simulink model "modellqrN1"  (R2023b)
settings: Solver=VariableStepAuto  StartTime=0.0  StopTime=1000  FixedStep=0.0001  MaxStep=1  MinStep=0.1  RelTol=1e-3
values from neighbouring files (symbols this model uses):
  g_ = 9.81    [main.m]
  h1_ = 0.15    [main.m]
  h2_ = (a^2*h1_)/(b^2)    [main.m]
  K = lqr(A,B,Q,R)    [main.m]
  N = 1/([0 1] *(-inv(A-B.*K'))* B)    [main.m]
  p1_ = 0.85    [main.m]
  p2_ = 0.95    [main.m]
  q0_ = a*sqrt(h1_)    [main.m]
  s1_ = 0.083    [main.m]
  S1_ = 2*pi*R1_*h1_ + 2*pi*R1_^2    (= 27.0176968209)    [main.m]
  s2_ = 0.083    [main.m]
  S2_ = 2*pi*R2_*h2_ + 2*pi*R2_^2    [main.m]
settings Model: Creator=ralex  LastModifiedBy=ralex

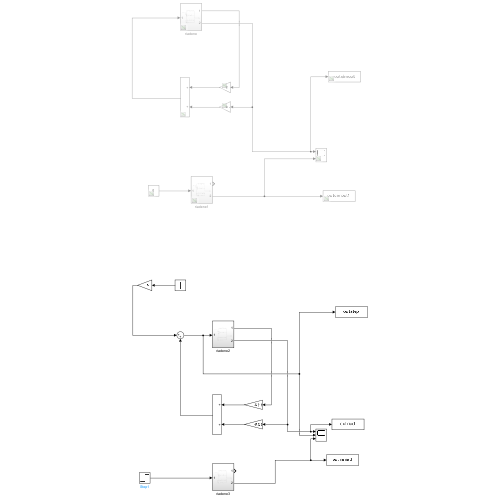
[thumbnail: Simulink's stored preview of the top-level diagram]
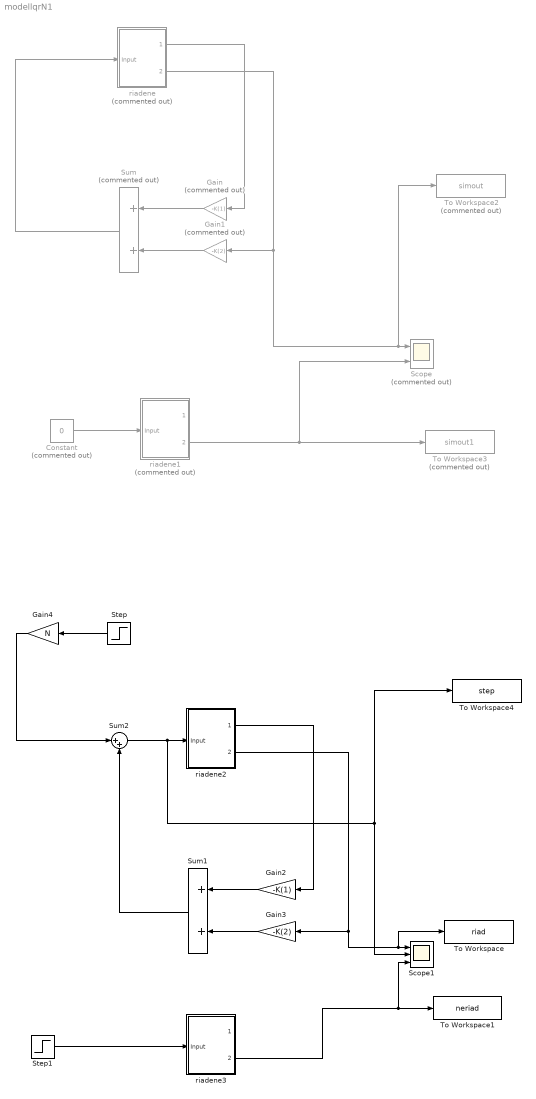
== system modellqrN1 ==
  Constant : Constant  Commented=on  Value=0
  Gain : Gain  Commented=on  Gain=-K(1)
  Gain1 : Gain  Commented=on  Gain=-K(2)
  Gain2 : Gain  Gain=-K(1)
  Gain3 : Gain  Gain=-K(2)
  Gain4 : Gain  Gain=N
  Scope : Scope  Commented=on  NumInputPorts=2
  Scope1 : Scope  NumInputPorts=3
  Step : Step  Time=100  After=h2_  SampleTime=0
  Step1 : Step  Time=100  After=q0_  SampleTime=0
  Sum : Sum  Commented=on
  Sum1 : Sum
  Sum2 : Sum  Inputs=|++
  To Workspace : ToWorkspace  VariableName=riad  SaveFormat=Timeseries  SampleTime=-1
  To Workspace1 : ToWorkspace  VariableName=neriad  SaveFormat=Timeseries  SampleTime=-1
  To Workspace2 : ToWorkspace  Commented=on  VariableName=simout  SaveFormat=Timeseries  SampleTime=-1
  To Workspace3 : ToWorkspace  Commented=on  VariableName=simout1  SaveFormat=Timeseries  SampleTime=-1
  To Workspace4 : ToWorkspace  VariableName=step  SaveFormat=Timeseries  SampleTime=-1
  riadene : Subsystem  Commented=on
  riadene1 : Subsystem  Commented=on
  riadene2 : Subsystem
  riadene3 : Subsystem
  wires:
  riadene/2(Output) -> To Workspace2/1, Scope/1, Gain1/1
  riadene/1(Output1) -> Gain/1
  Gain1/1 -> Sum/2
  Gain/1 -> Sum/1
  Sum/1 -> riadene/1(Input)
  Constant/1 -> riadene1/1(Input)
  riadene1/2(Output) -> To Workspace3/1, Scope/2
  Gain2/1 -> Sum1/1
  Gain3/1 -> Sum1/2
  Step/1 -> Gain4/1
  Sum2/1 -> To Workspace4/1, Scope1/2, riadene2/1(Input)
  Sum1/1 -> Sum2/2
  Gain4/1 -> Sum2/1
  riadene2/2(Output) -> To Workspace/1, Scope1/1, Gain3/1
  riadene2/1(Output1) -> Gain2/1
  riadene3/2(Output) -> Scope1/3, To Workspace1/1
  Step1/1 -> riadene3/1(Input)

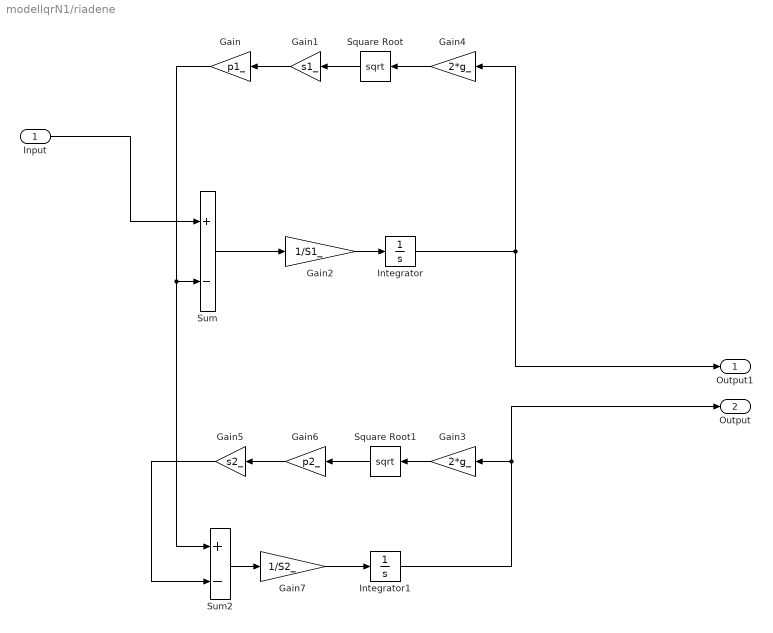
== system modellqrN1/riadene ==
  Input : Inport
  Gain : Gain  Gain=p1_
  Gain1 : Gain  Gain=s1_
  Gain2 : Gain  Gain=1/S1_
  Gain3 : Gain  Gain=2*g_
  Gain4 : Gain  Gain=2*g_
  Gain5 : Gain  Gain=s2_
  Gain6 : Gain  Gain=p2_
  Gain7 : Gain  Gain=1/S2_
  Integrator : Integrator  InitialCondition=h1_
  Integrator1 : Integrator  InitialCondition=h2_
  Square Root : Sqrt
  Square Root1 : Sqrt
  Sum : Sum  Inputs=+-
  Sum2 : Sum  Inputs=+-
  Output1 : Outport
  Output : Outport  Port=2
  wires:
  Gain/1 -> Sum/2, Sum2/1
  Gain1/1 -> Gain/1
  Input/1 -> Sum/1
  Integrator/1 -> Output1/1, Gain4/1
  Square Root/1 -> Gain1/1
  Gain4/1 -> Square Root/1
  Gain5/1 -> Sum2/2
  Sum/1 -> Gain2/1
  Integrator1/1 -> Output/1, Gain3/1
  Gain6/1 -> Gain5/1
  Square Root1/1 -> Gain6/1
  Gain3/1 -> Square Root1/1
  Sum2/1 -> Gain7/1
  Gain2/1 -> Integrator/1
  Gain7/1 -> Integrator1/1

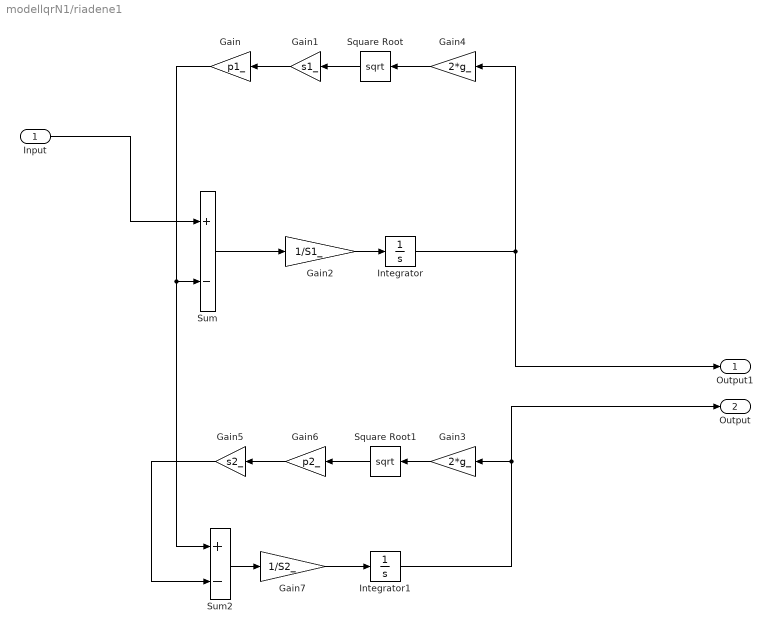
== system modellqrN1/riadene1 ==
  Input : Inport
  Gain : Gain  Gain=p1_
  Gain1 : Gain  Gain=s1_
  Gain2 : Gain  Gain=1/S1_
  Gain3 : Gain  Gain=2*g_
  Gain4 : Gain  Gain=2*g_
  Gain5 : Gain  Gain=s2_
  Gain6 : Gain  Gain=p2_
  Gain7 : Gain  Gain=1/S2_
  Integrator : Integrator  InitialCondition=h1_
  Integrator1 : Integrator  InitialCondition=h2_
  Square Root : Sqrt
  Square Root1 : Sqrt
  Sum : Sum  Inputs=+-
  Sum2 : Sum  Inputs=+-
  Output1 : Outport
  Output : Outport  Port=2
  wires:
  Gain/1 -> Sum/2, Sum2/1
  Gain1/1 -> Gain/1
  Input/1 -> Sum/1
  Integrator/1 -> Output1/1, Gain4/1
  Square Root/1 -> Gain1/1
  Gain4/1 -> Square Root/1
  Gain5/1 -> Sum2/2
  Sum/1 -> Gain2/1
  Integrator1/1 -> Output/1, Gain3/1
  Gain6/1 -> Gain5/1
  Square Root1/1 -> Gain6/1
  Gain3/1 -> Square Root1/1
  Sum2/1 -> Gain7/1
  Gain2/1 -> Integrator/1
  Gain7/1 -> Integrator1/1

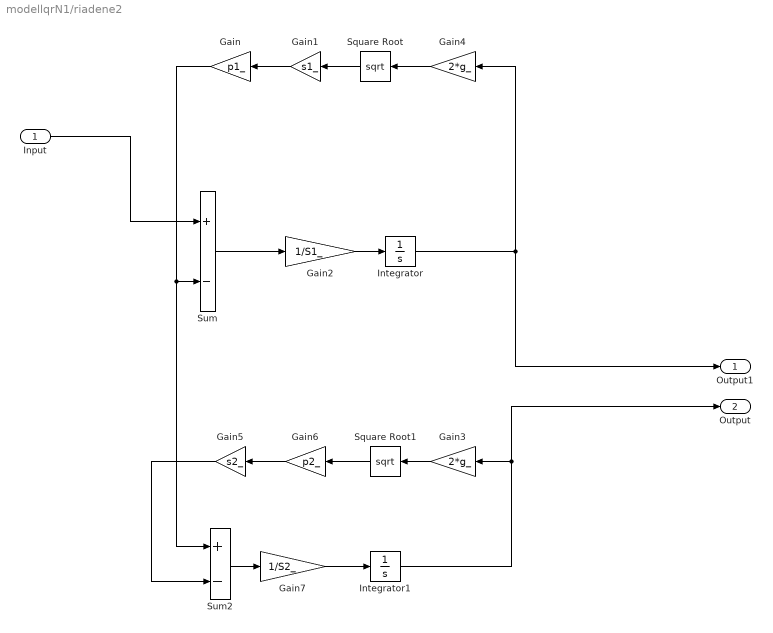
== system modellqrN1/riadene2 ==
  Input : Inport
  Gain : Gain  Gain=p1_
  Gain1 : Gain  Gain=s1_
  Gain2 : Gain  Gain=1/S1_
  Gain3 : Gain  Gain=2*g_
  Gain4 : Gain  Gain=2*g_
  Gain5 : Gain  Gain=s2_
  Gain6 : Gain  Gain=p2_
  Gain7 : Gain  Gain=1/S2_
  Integrator : Integrator
  Integrator1 : Integrator
  Square Root : Sqrt
  Square Root1 : Sqrt
  Sum : Sum  Inputs=+-
  Sum2 : Sum  Inputs=+-
  Output1 : Outport
  Output : Outport  Port=2
  wires:
  Gain/1 -> Sum/2, Sum2/1
  Gain1/1 -> Gain/1
  Input/1 -> Sum/1
  Integrator/1 -> Output1/1, Gain4/1
  Square Root/1 -> Gain1/1
  Gain4/1 -> Square Root/1
  Gain5/1 -> Sum2/2
  Sum/1 -> Gain2/1
  Integrator1/1 -> Output/1, Gain3/1
  Gain6/1 -> Gain5/1
  Square Root1/1 -> Gain6/1
  Gain3/1 -> Square Root1/1
  Sum2/1 -> Gain7/1
  Gain2/1 -> Integrator/1
  Gain7/1 -> Integrator1/1

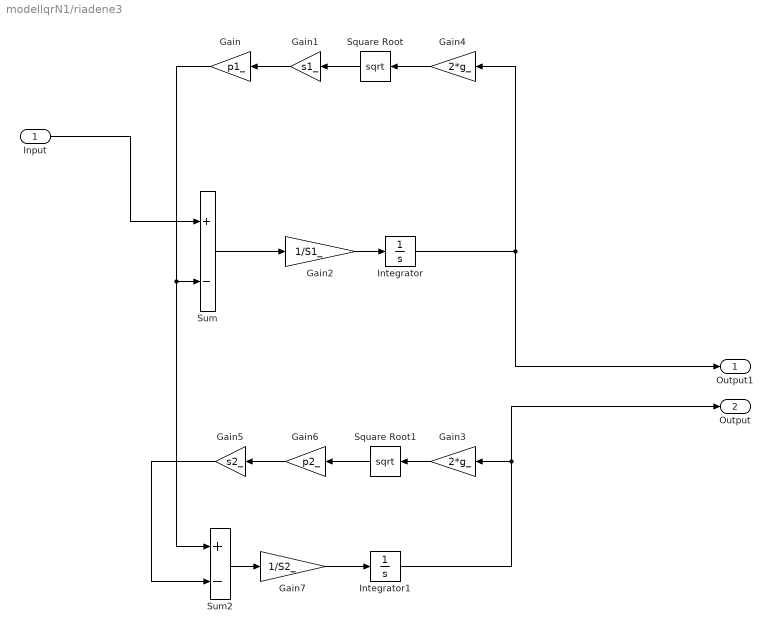
== system modellqrN1/riadene3 ==
  Input : Inport
  Gain : Gain  Gain=p1_
  Gain1 : Gain  Gain=s1_
  Gain2 : Gain  Gain=1/S1_
  Gain3 : Gain  Gain=2*g_
  Gain4 : Gain  Gain=2*g_
  Gain5 : Gain  Gain=s2_
  Gain6 : Gain  Gain=p2_
  Gain7 : Gain  Gain=1/S2_
  Integrator : Integrator
  Integrator1 : Integrator
  Square Root : Sqrt
  Square Root1 : Sqrt
  Sum : Sum  Inputs=+-
  Sum2 : Sum  Inputs=+-
  Output1 : Outport
  Output : Outport  Port=2
  wires:
  Gain/1 -> Sum/2, Sum2/1
  Gain1/1 -> Gain/1
  Input/1 -> Sum/1
  Integrator/1 -> Output1/1, Gain4/1
  Square Root/1 -> Gain1/1
  Gain4/1 -> Square Root/1
  Gain5/1 -> Sum2/2
  Sum/1 -> Gain2/1
  Integrator1/1 -> Output/1, Gain3/1
  Gain6/1 -> Gain5/1
  Square Root1/1 -> Gain6/1
  Gain3/1 -> Square Root1/1
  Sum2/1 -> Gain7/1
  Gain2/1 -> Integrator/1
  Gain7/1 -> Integrator1/1
